simulink model "cacc_platoon"  (R2026a)
settings: Solver=ode4  StartTime=0  StopTime=Tend  FixedStep=dt
undefined symbols (not defined in the file or in its folder): a0_amp, a0_dur, a0_omega, a0_t0, a_init, d, gamma_rep, hw, ka, kp, kv, noise_bias, noise_K, PredSel, seed_vec, tau_inv, ts_noise, v_init, v_ss, x0_lead, x_init

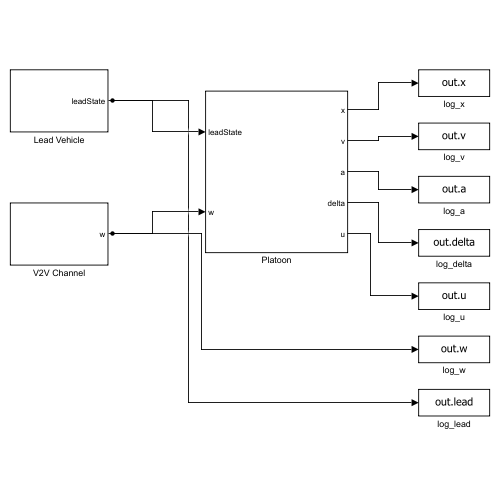
[thumbnail: Simulink's stored preview of the top-level diagram]
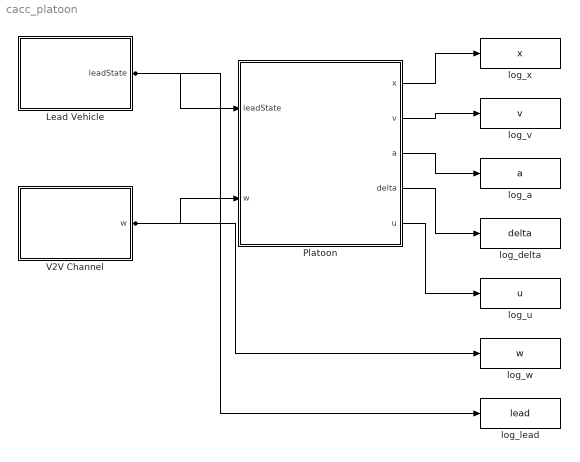
== system cacc_platoon ==
  Lead Vehicle : Subsystem
  Platoon : Subsystem
  V2V Channel : Subsystem
  log_a : ToWorkspace  VariableName=a  SaveFormat=Timeseries  SampleTime=-1
  log_delta : ToWorkspace  VariableName=delta  SaveFormat=Timeseries  SampleTime=-1
  log_lead : ToWorkspace  VariableName=lead  SaveFormat=Timeseries  SampleTime=-1
  log_u : ToWorkspace  VariableName=u  SaveFormat=Timeseries  SampleTime=-1
  log_v : ToWorkspace  VariableName=v  SaveFormat=Timeseries  SampleTime=-1
  log_w : ToWorkspace  VariableName=w  SaveFormat=Timeseries  SampleTime=-1
  log_x : ToWorkspace  VariableName=x  SaveFormat=Timeseries  SampleTime=-1
  wires:
  Lead Vehicle/1(leadState) -> Platoon/1(leadState), log_lead/1
  V2V Channel/1(w) -> Platoon/2(w), log_w/1
  Platoon/1(x) -> log_x/1
  Platoon/2(v) -> log_v/1
  Platoon/3(a) -> log_a/1
  Platoon/4(delta) -> log_delta/1
  Platoon/5(u) -> log_u/1

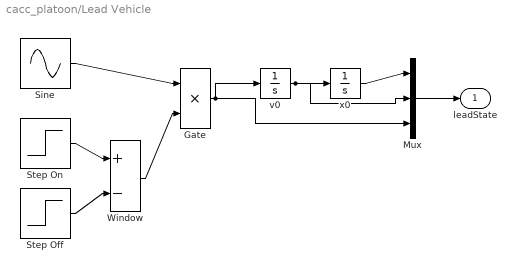
== system cacc_platoon/Lead Vehicle ==
  Gate : Product
  Mux : Mux  Inputs=3
  Sine : Sin  Amplitude=a0_amp  Frequency=a0_omega  Phase=-a0_omega*a0_t0  SampleTime=0
  Step Off : Step  Time=a0_t0+a0_dur  SampleTime=0
  Step On : Step  Time=a0_t0  SampleTime=0
  Window : Sum  Inputs=+-
  v0 : Integrator  InitialCondition=v_ss
  x0 : Integrator  InitialCondition=x0_lead
  leadState : Outport
  wires:
  Step On/1 -> Window/1
  Step Off/1 -> Window/2
  Sine/1 -> Gate/1
  Window/1 -> Gate/2
  Gate/1 -> v0/1, Mux/3
  v0/1 -> x0/1, Mux/2
  x0/1 -> Mux/1
  Mux/1 -> leadState/1

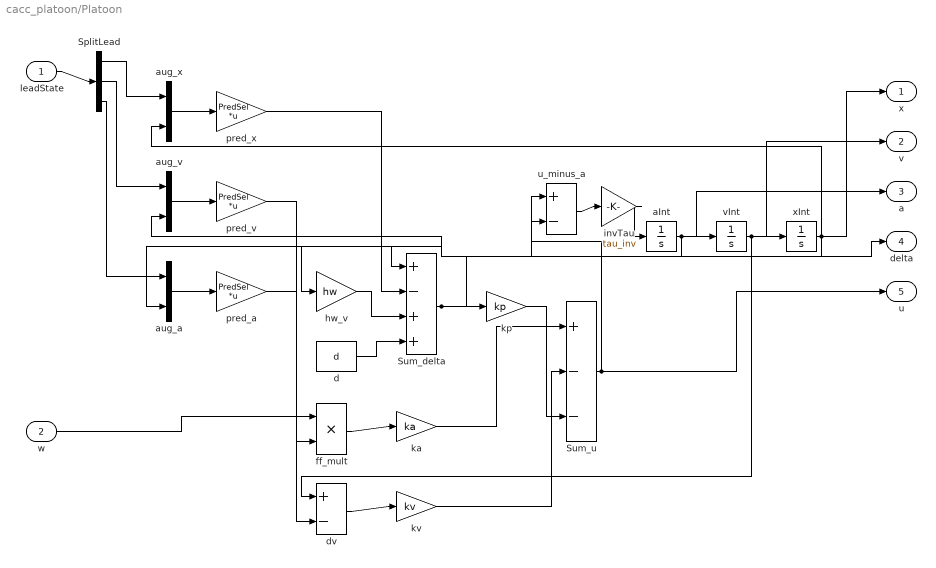
== system cacc_platoon/Platoon ==
  leadState : Inport
  w : Inport  Port=2
  SplitLead : Demux  Outputs=3
  Sum_delta : Sum  Inputs=+-++
  Sum_u : Sum  Inputs=+--
  aInt : Integrator  InitialCondition=a_init
  aug_a : Mux  Inputs=2
  aug_v : Mux  Inputs=2
  aug_x : Mux  Inputs=2
  d : Constant  Value=d
  dv : Sum  Inputs=+-
  ff_mult : Product
  hw_v : Gain  Gain=hw
  invTau : Gain  Gain=tau_inv
  ka : Gain  Gain=ka
  kp : Gain  Gain=kp
  kv : Gain  Gain=kv
  pred_a : Gain  Gain=PredSel  Multiplication=Matrix(K*u)
  pred_v : Gain  Gain=PredSel  Multiplication=Matrix(K*u)
  pred_x : Gain  Gain=PredSel  Multiplication=Matrix(K*u)
  u_minus_a : Sum  Inputs=+-
  vInt : Integrator  InitialCondition=v_init
  xInt : Integrator  InitialCondition=x_init
  x : Outport
  v : Outport  Port=2
  a : Outport  Port=3
  delta : Outport  Port=4
  u : Outport  Port=5
  wires:
  SplitLead/1 -> aug_x/1
  aug_x/1 -> pred_x/1
  SplitLead/2 -> aug_v/1
  aug_v/1 -> pred_v/1
  SplitLead/3 -> aug_a/1
  aug_a/1 -> pred_a/1
  leadState/1 -> SplitLead/1
  xInt/1 -> Sum_delta/1, x/1, aug_x/2
  pred_x/1 -> Sum_delta/2
  hw_v/1 -> Sum_delta/3
  d/1 -> Sum_delta/4
  vInt/1 -> hw_v/1, dv/1, xInt/1, v/1, aug_v/2
  w/1 -> ff_mult/1
  pred_a/1 -> ff_mult/2
  ff_mult/1 -> ka/1
  pred_v/1 -> dv/2
  dv/1 -> kv/1
  Sum_delta/1 -> kp/1, delta/1
  ka/1 -> Sum_u/1
  kv/1 -> Sum_u/2
  kp/1 -> Sum_u/3
  Sum_u/1 -> u_minus_a/1, u/1
  aInt/1 -> u_minus_a/2, vInt/1, a/1, aug_a/2
  u_minus_a/1 -> invTau/1
  invTau/1 -> aInt/1

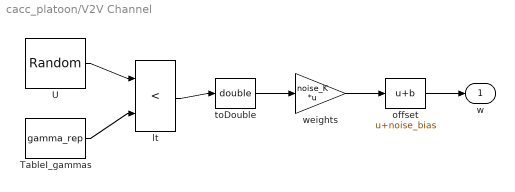
== system cacc_platoon/V2V Channel ==
  TableI_gammas : Constant  Value=gamma_rep
  U : UniformRandomNumber  Minimum=0  Seed=seed_vec  SampleTime=ts_noise
  lt : RelationalOperator  Operator=<  OutDataTypeStr=boolean  RndMeth=Simplest  InputSameDT=off
  offset : Bias  Bias=noise_bias  SaturateOnIntegerOverflow=off
  toDouble : DataTypeConversion  OutDataTypeStr=double  SaturateOnIntegerOverflow=off  RndMeth=Floor
  weights : Gain  Gain=noise_K  Multiplication=Matrix(K*u)
  w : Outport
  wires:
  U/1 -> lt/1
  TableI_gammas/1 -> lt/2
  lt/1 -> toDouble/1
  toDouble/1 -> weights/1
  weights/1 -> offset/1
  offset/1 -> w/1
